simulink model "line_follower"  (R2020a)
settings: Solver=VariableStepAuto  StartTime=0.0  StopTime=70  RelTol=1e-3
InitFcn:
  | matlab_init
undefined symbols (not defined in the file or in its folder): A, A_double, A_s_double, A_s_single, A_single, Aaileron, Aelevator, Arudder, Athrust, B, B_double, B_s_double, B_s_single, B_single, Baileron, Belevator, Brudder, Bthrust, C, C_double, C_P, C_rollpitch, C_single, C_T, C_yaw, Caileron, Celevator, Crudder, Cthrust, D, D_double, D_single, Daileron, Delevator, DiscIntNeverNeededParam, Discrete, Drudder, Dthrust, g, I_flip, J, Jinv, K_a, K_e, K_r, K_t, L_double, L_single, measurement_noise, MotorMix, process_noise, Prop_H, q_single, r_single, tau2, Thrust_Sum, Time, trim_input, trim_state, Ts ... (+1)
libraries: simulink x5, ctrlSharedLib x5, vrlib x3, dspmtrx3 x1
(part 2 of 2)

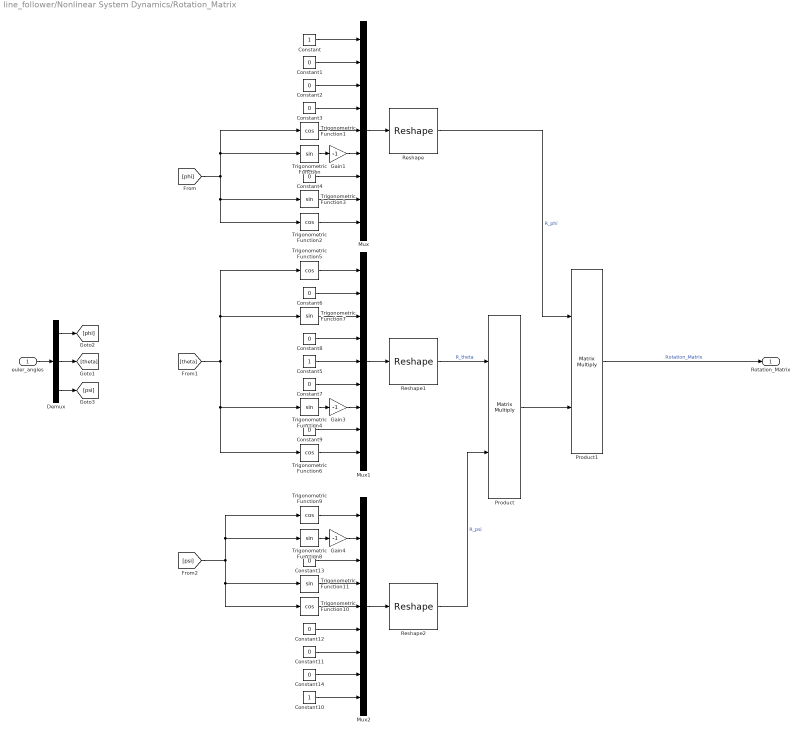
== system line_follower/Nonlinear System Dynamics/Rotation_Matrix ==
  "euler_angles " : Inport
  Constant : Constant
  Constant{1..4,6..9,11..14} (12 alike) : Constant  Value=0
  Constant10 : Constant
  Constant5 : Constant
  Demux : Demux  Outputs=3
  Gain1 : Gain  Gain=-1
  Gain3 : Gain  Gain=-1
  Gain4 : Gain  Gain=-1
  Mux : Mux  Inputs=9
  Mux1 : Mux  Inputs=9
  Mux2 : Mux  Inputs=9
  Product : Product  Multiplication=Matrix(*)
  Product1 : Product  Multiplication=Matrix(*)
  Reshape : Reshape  OutputDimensionality=Customize  OutputDimensions=[3,3]
  Reshape1 : Reshape  OutputDimensionality=Customize  OutputDimensions=[3,3]
  Reshape2 : Reshape  OutputDimensionality=Customize  OutputDimensions=[3,3]
  Trigonometric Function{,3..4,7..8,11} (6 alike) : Trigonometry
  Trigonometric Function{1..2,5..6,9..10} (6 alike) : Trigonometry  Operator=cos
  Rotation_Matrix : Outport
  wires:
  Constant9/1 -> Mux1/8
  Constant11/1 -> Mux2/7
  Trigonometric Function1/1 -> Mux/5
  Trigonometric Function3/1 -> Mux/8
  Constant5/1 -> Mux1/5
  Trigonometric Function7/1 -> Mux1/3
  Reshape/1 -> Product1/1  "R_phi"
  Mux1/1 -> Reshape1/1
  Trigonometric Function8/1 -> Gain4/1
  Constant7/1 -> Mux1/6
  Trigonometric Function2/1 -> Mux/9
  [phi] -> Trigonometric Function2/1, Trigonometric Function3/1, Trigonometric Function1/1, Trigonometric Function/1
  Trigonometric Function6/1 -> Mux1/9
  Constant12/1 -> Mux2/6
  Trigonometric Function4/1 -> Gain3/1
  [theta] -> Trigonometric Function7/1, Trigonometric Function5/1, Trigonometric Function4/1, Trigonometric Function6/1
  Reshape2/1 -> Product/2  "R_psi"
  Trigonometric Function/1 -> Gain1/1
  Product/1 -> Product1/2
  Trigonometric Function5/1 -> Mux1/1
  Trigonometric Function9/1 -> Mux2/1
  Mux/1 -> Reshape/1
  Constant/1 -> Mux/1
  Constant3/1 -> Mux/4
  Constant6/1 -> Mux1/2
  Mux2/1 -> Reshape2/1
  Constant2/1 -> Mux/3
  Constant1/1 -> Mux/2
  [psi] -> Trigonometric Function11/1, Trigonometric Function10/1, Trigonometric Function9/1, Trigonometric Function8/1
  Constant8/1 -> Mux1/4
  Constant4/1 -> Mux/7
  Constant13/1 -> Mux2/3
  Trigonometric Function11/1 -> Mux2/4
  Constant10/1 -> Mux2/9
  Reshape1/1 -> Product/1  "R_theta"
  Constant14/1 -> Mux2/8
  Trigonometric Function10/1 -> Mux2/5
  Product1/1 -> Rotation_Matrix/1  "Rotation_Matrix"
  Demux/3 -> [psi]
  Demux/2 -> [theta]
  "euler_angles "/1 -> Demux/1
  Demux/1 -> [phi]
  Gain3/1 -> Mux1/7
  Gain1/1 -> Mux/6
  Gain4/1 -> Mux2/2

== system line_follower/Toggle Controller/Hover ==
  Mux : Mux  Inputs=9
  p : Constant  Value=0
  phi : Constant  Value=0
  q : Constant  Value=0
  r : Constant  Value=0
  theta : Constant  Value=0
  u : Constant  Value=0
  v : Constant  Value=0
  w : Constant  Value=0
  z : Constant  Value=1.5
  Out1 : Outport
  wires:
  theta/1 -> Mux/8
  u/1 -> Mux/1
  p/1 -> Mux/5
  r/1 -> Mux/7
  z/1 -> Mux/4
  q/1 -> Mux/6
  phi/1 -> Mux/9
  w/1 -> Mux/3
  v/1 -> Mux/2
  Mux/1 -> Out1/1

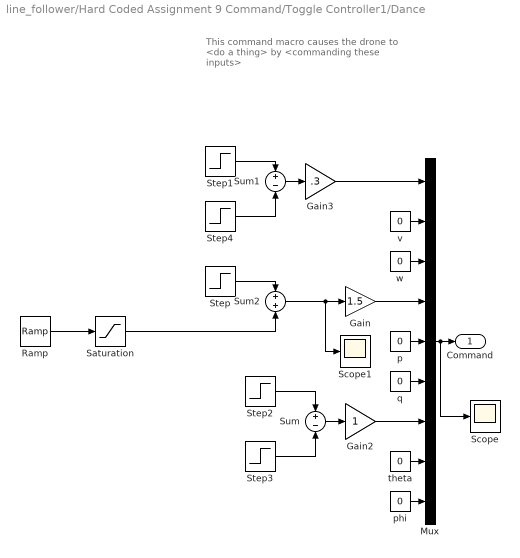
== system line_follower/Hard Coded Assignment 9 Command/Toggle Controller1/Dance ==
  note: This command macro causes the drone to <do a thing> by <commanding these inputs>
  Gain : Gain  Gain=1.5
  Gain2 : Gain
  Gain3 : Gain  Gain=.3
  Mux : Mux  Inputs=9
  Ramp : simulink/Sources/Ramp  slope=-.3  start=17  InitialOutput=0
  Saturation : Saturate  UpperLimit=1  LowerLimit=-1
  Scope : Scope
  Scope1 : Scope
  Step : Step  SampleTime=0
  Step1 : Step  Time=4  SampleTime=0
  Step2 : Step  Time=7  SampleTime=0
  Step3 : Step  Time=13.5  SampleTime=0
  Step4 : Step  Time=13.5  SampleTime=0
  Sum : Sum  Inputs=+-
  Sum1 : Sum  Inputs=+-
  Sum2 : Sum
  p : Constant  Value=0
  phi : Constant  Value=0
  q : Constant  Value=0
  theta : Constant  Value=0
  v : Constant  Value=0
  w : Constant  Value=0
  Command : Outport
  wires:
  Mux/1 -> Scope/1, Command/1
  theta/1 -> Mux/8
  p/1 -> Mux/5
  q/1 -> Mux/6
  v/1 -> Mux/2
  phi/1 -> Mux/9
  w/1 -> Mux/3
  Gain/1 -> Mux/4
  Step1/1 -> Sum1/1
  Step2/1 -> Sum/1
  Step3/1 -> Sum/2
  Sum/1 -> Gain2/1
  Gain2/1 -> Mux/7
  Sum1/1 -> Gain3/1
  Step4/1 -> Sum1/2
  Gain3/1 -> Mux/1
  Step/1 -> Sum2/1
  Sum2/1 -> Scope1/1, Gain/1
  Ramp/1 -> Saturation/1
  Saturation/1 -> Sum2/2

== system line_follower/Hard Coded Elevator Flip/Toggle Controller1/Hover ==
  Mux : Mux  Inputs=9
  p : Constant  Value=0
  phi : Constant  Value=0
  q : Constant  Value=0
  r : Constant  Value=0
  theta : Constant  Value=0
  u : Constant  Value=0
  v : Constant  Value=0
  w : Constant  Value=0
  z : Constant  Value=1.5
  Out1 : Outport
  wires:
  Mux/1 -> Out1/1
  v/1 -> Mux/2
  w/1 -> Mux/3
  phi/1 -> Mux/9
  q/1 -> Mux/6
  z/1 -> Mux/4
  r/1 -> Mux/7
  p/1 -> Mux/5
  u/1 -> Mux/1
  theta/1 -> Mux/8

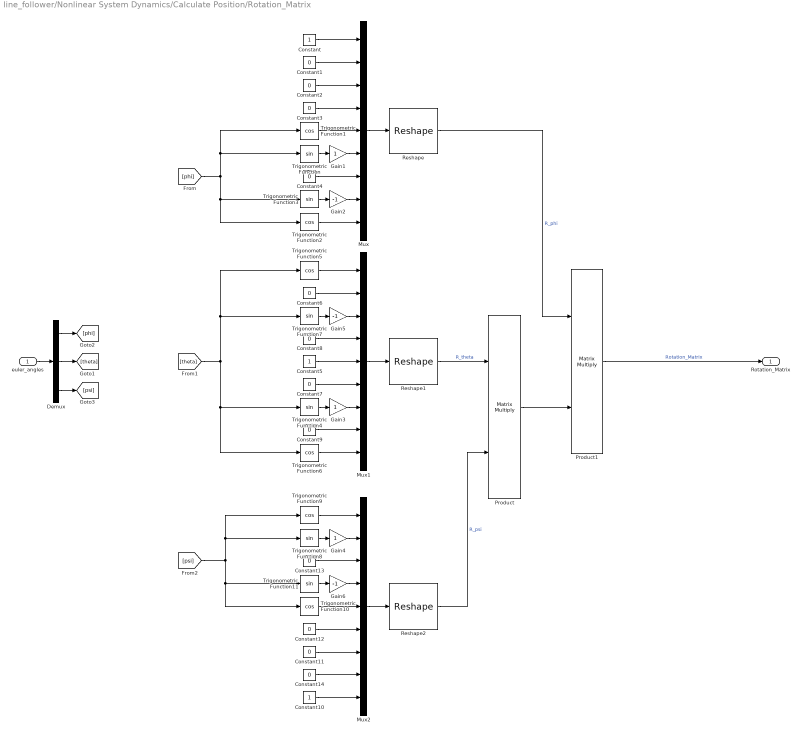
== system line_follower/Nonlinear System Dynamics/Calculate Position/Rotation_Matrix ==
  "euler_angles " : Inport
  Constant : Constant
  Constant{1..4,6..9,11..14} (12 alike) : Constant  Value=0
  Constant10 : Constant
  Constant5 : Constant
  Demux : Demux  Outputs=3
  Gain1 : Gain
  Gain2 : Gain  Gain=-1
  Gain3 : Gain
  Gain4 : Gain
  Gain5 : Gain  Gain=-1
  Gain6 : Gain  Gain=-1
  Mux : Mux  Inputs=9
  Mux1 : Mux  Inputs=9
  Mux2 : Mux  Inputs=9
  Product : Product  Multiplication=Matrix(*)
  Product1 : Product  Multiplication=Matrix(*)
  Reshape : Reshape  OutputDimensionality=Customize  OutputDimensions=[3,3]
  Reshape1 : Reshape  OutputDimensionality=Customize  OutputDimensions=[3,3]
  Reshape2 : Reshape  OutputDimensionality=Customize  OutputDimensions=[3,3]
  Trigonometric Function{,3..4,7..8,11} (6 alike) : Trigonometry
  Trigonometric Function{1..2,5..6,9..10} (6 alike) : Trigonometry  Operator=cos
  Rotation_Matrix : Outport
  wires:
  Constant9/1 -> Mux1/8
  Constant11/1 -> Mux2/7
  Trigonometric Function1/1 -> Mux/5
  Trigonometric Function3/1 -> Gain2/1
  Constant5/1 -> Mux1/5
  Trigonometric Function7/1 -> Gain5/1
  Reshape/1 -> Product1/1  "R_phi"
  Mux1/1 -> Reshape1/1
  Trigonometric Function8/1 -> Gain4/1
  Constant7/1 -> Mux1/6
  Trigonometric Function2/1 -> Mux/9
  [phi] -> Trigonometric Function2/1, Trigonometric Function3/1, Trigonometric Function1/1, Trigonometric Function/1
  Trigonometric Function6/1 -> Mux1/9
  Constant12/1 -> Mux2/6
  Trigonometric Function4/1 -> Gain3/1
  [theta] -> Trigonometric Function7/1, Trigonometric Function5/1, Trigonometric Function4/1, Trigonometric Function6/1
  Reshape2/1 -> Product/2  "R_psi"
  Trigonometric Function/1 -> Gain1/1
  Product/1 -> Product1/2
  Trigonometric Function5/1 -> Mux1/1
  Trigonometric Function9/1 -> Mux2/1
  Mux/1 -> Reshape/1
  Constant/1 -> Mux/1
  Constant3/1 -> Mux/4
  Constant6/1 -> Mux1/2
  Mux2/1 -> Reshape2/1
  Constant2/1 -> Mux/3
  Constant1/1 -> Mux/2
  [psi] -> Trigonometric Function11/1, Trigonometric Function10/1, Trigonometric Function9/1, Trigonometric Function8/1
  Constant8/1 -> Mux1/4
  Constant4/1 -> Mux/7
  Constant13/1 -> Mux2/3
  Trigonometric Function11/1 -> Gain6/1
  Constant10/1 -> Mux2/9
  Reshape1/1 -> Product/1  "R_theta"
  Constant14/1 -> Mux2/8
  Trigonometric Function10/1 -> Mux2/5
  Product1/1 -> Rotation_Matrix/1  "Rotation_Matrix"
  Demux/3 -> [psi]
  Demux/2 -> [theta]
  "euler_angles "/1 -> Demux/1
  Demux/1 -> [phi]
  Gain3/1 -> Mux1/7
  Gain1/1 -> Mux/6
  Gain4/1 -> Mux2/2
  Gain2/1 -> Mux/8
  Gain5/1 -> Mux1/3
  Gain6/1 -> Mux2/4

== system line_follower/Nonlinear System Dynamics/Calculate Velocity/Calculate_Thrust ==
  note: $F_{T} = \sum_{i=1}^4[0;0;C_{T}.*n.^2]$
  n : Inport
  Constant15 : Constant  Value=C_T(1)
  Constant16 : Constant  Value=2
  Gain4 : Gain  Gain=Thrust_Sum  Multiplication=Matrix(K*u)
      settings: AttributesFormatString=%<Gain>
  Gain5 : Gain  Gain=C_T(2)
  Power : Math  Operator=pow  SaturateOnIntegerOverflow=on
  Product2 : Product
  Sum1 : Sum  Inputs=++|
  F_T : Outport
  wires:
  Constant15/1 -> Sum1/1
  Gain4/1 -> F_T/1  "F_T"
  n/1 -> Power/1, Gain5/1
  Power/1 -> Product2/2  "props squared"
  Gain5/1 -> Sum1/2
  Sum1/1 -> Product2/1
  Product2/1 -> Gain4/1
  Constant16/1 -> Power/2

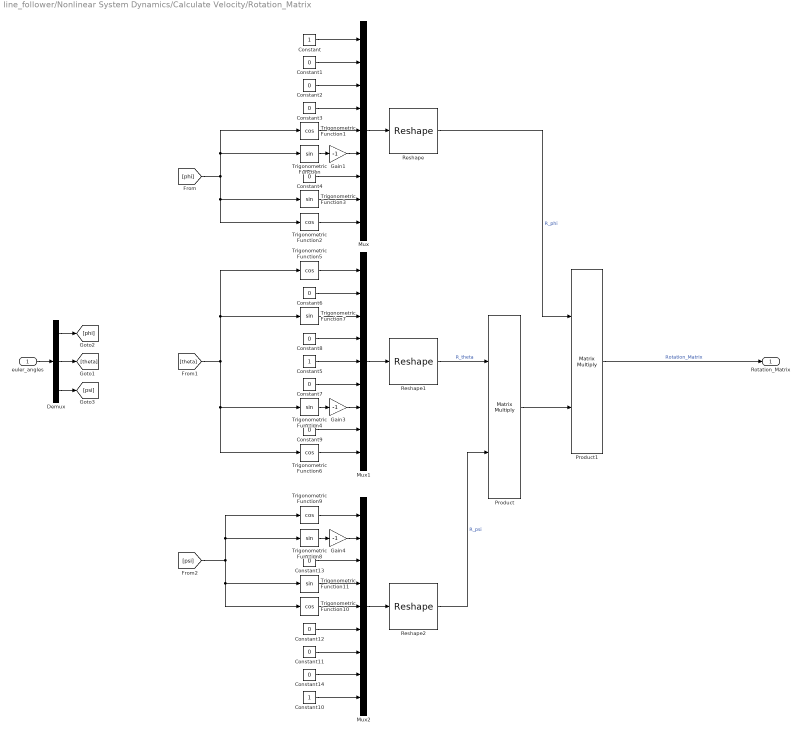
== system line_follower/Nonlinear System Dynamics/Calculate Velocity/Rotation_Matrix ==
  "euler_angles " : Inport
  Constant : Constant
  Constant{1..4,6..9,11..14} (12 alike) : Constant  Value=0
  Constant10 : Constant
  Constant5 : Constant
  Demux : Demux  Outputs=3
  Gain1 : Gain  Gain=-1
  Gain3 : Gain  Gain=-1
  Gain4 : Gain  Gain=-1
  Mux : Mux  Inputs=9
  Mux1 : Mux  Inputs=9
  Mux2 : Mux  Inputs=9
  Product : Product  Multiplication=Matrix(*)
  Product1 : Product  Multiplication=Matrix(*)
  Reshape : Reshape  OutputDimensionality=Customize  OutputDimensions=[3,3]
  Reshape1 : Reshape  OutputDimensionality=Customize  OutputDimensions=[3,3]
  Reshape2 : Reshape  OutputDimensionality=Customize  OutputDimensions=[3,3]
  Trigonometric Function{,3..4,7..8,11} (6 alike) : Trigonometry
  Trigonometric Function{1..2,5..6,9..10} (6 alike) : Trigonometry  Operator=cos
  Rotation_Matrix : Outport
  wires:
  Constant9/1 -> Mux1/8
  Constant11/1 -> Mux2/7
  Trigonometric Function1/1 -> Mux/5
  Trigonometric Function3/1 -> Mux/8
  Constant5/1 -> Mux1/5
  Trigonometric Function7/1 -> Mux1/3
  Reshape/1 -> Product1/1  "R_phi"
  Mux1/1 -> Reshape1/1
  Trigonometric Function8/1 -> Gain4/1
  Constant7/1 -> Mux1/6
  Trigonometric Function2/1 -> Mux/9
  [phi] -> Trigonometric Function2/1, Trigonometric Function3/1, Trigonometric Function1/1, Trigonometric Function/1
  Trigonometric Function6/1 -> Mux1/9
  Constant12/1 -> Mux2/6
  Trigonometric Function4/1 -> Gain3/1
  [theta] -> Trigonometric Function7/1, Trigonometric Function5/1, Trigonometric Function4/1, Trigonometric Function6/1
  Reshape2/1 -> Product/2  "R_psi"
  Trigonometric Function/1 -> Gain1/1
  Product/1 -> Product1/2
  Trigonometric Function5/1 -> Mux1/1
  Trigonometric Function9/1 -> Mux2/1
  Mux/1 -> Reshape/1
  Constant/1 -> Mux/1
  Constant3/1 -> Mux/4
  Constant6/1 -> Mux1/2
  Mux2/1 -> Reshape2/1
  Constant2/1 -> Mux/3
  Constant1/1 -> Mux/2
  [psi] -> Trigonometric Function11/1, Trigonometric Function10/1, Trigonometric Function9/1, Trigonometric Function8/1
  Constant8/1 -> Mux1/4
  Constant4/1 -> Mux/7
  Constant13/1 -> Mux2/3
  Trigonometric Function11/1 -> Mux2/4
  Constant10/1 -> Mux2/9
  Reshape1/1 -> Product/1  "R_theta"
  Constant14/1 -> Mux2/8
  Trigonometric Function10/1 -> Mux2/5
  Product1/1 -> Rotation_Matrix/1  "Rotation_Matrix"
  Demux/3 -> [psi]
  Demux/2 -> [theta]
  "euler_angles "/1 -> Demux/1
  Demux/1 -> [phi]
  Gain3/1 -> Mux1/7
  Gain1/1 -> Mux/6
  Gain4/1 -> Mux2/2

== matlab function line_follower/Control Design/Virtual Hough Transform Circle ==
  settings: updateMethod=DISCRETE  sampleTime=0.005
  data: y_cmd output; psi_cmd output; XY input
function [y_cmd, psi_cmd]= fcn(XY)

%% INIT X,Y to 0,2

x = XY(1);
y = XY(2);

path_rad = 2;

uav_rad = sqrt(x^2+y^2);
y_cmd = (uav_rad - path_rad);

path_angle = atan2(x,y);

if path_angle < -0.1
    path_angle = path_angle + 2*pi;
end

psi_cmd = (path_angle);

== matlab function line_follower/Drone Visualization ==
  data: T input
function drone_visualization(T)

%% /// IMPORTANT ///
%T is array that hold states
%ZED is pointing downwards
%MAKE A MATLAB FUNCTION BLOCK IN SIMULINK
%PASS IN THE NED STATES AND EULER ANGLES
%ADJUST THE STATES AS NECESSARY
%the drone is .18 meters by .18 meters

%the simulation will run MUCH slower while running the visualization
%you can comment out the function block to run the simulation quicker

%% constants
d = .18/2;
c1 = [d; d; 0]; %motor coordinates compared to center of drone
c2 = [d; -d; 0];
c3 = -c1;
c4 = -c2;

    %% adjust indices to get [X; Y; Z] and phi, theta, psi
    XYZ =  [T(1); ...
            T(2); ...
           -T(3)];
    phi =   T(7);
    theta = T(8);
    psi =   T(9);
    %%Defining rotation matrices
    Rx = [1 0 0; 0 cos(theta) sin(theta); 0 -sin(theta) cos(theta)];
    Ry = [cos(phi) 0 -sin(phi); 0 1 0; sin(phi) 0 cos(phi)];
    Rz = [cos(psi) sin(psi) 0; -sin(psi) cos(psi) 0; 0 0 1];
    b1 = Rz*Ry*Rx*c1;
    b2 = Rz*Ry*Rx*c2;
    b3 = Rz*Ry*Rx*c3;
    b4 = Rz*Ry*Rx*c4;
    m1 = XYZ + b1;
    m2 = XYZ + b2;
    m3 = XYZ + b3;
    m4 = XYZ + b4;
    P1 = [m1 m3];
    P2 = [m2 m4];
    P3 = [m1 m2];
    P4 = [m3 m4];

    %%displaying the drone
    plot3(P1(1,:),P1(2,:),P1(3,:),'k-', 'linewidth', 2);
    axis([-3 3 -3 3 -0 3]);
    xlabel('X Axis [Meters]')
    ylabel('Y Axis [Meters]')
    zlabel('Height [Meters]')
    hold on;
    grid on;
    plot3(P2(1,:),P2(2,:),P2(3,:),'k-', 'linewidth', 2);
    plot3(P3(1,:),P3(2,:),P3(3,:),'ob', 'linewidth', 1);
    plot3(P4(1,:),P4(2,:),P4(3,:),'ok', 'linewidth', 1);
    hold off
end

== matlab function line_follower/Control Design/Virtual Hough Transform Line ==
  settings: sampleTime=0.05
  data: y_cmd output; psi_cmd output; XY input
function [y_cmd, psi_cmd]= fcn(XY)

%% INIT X,Y to 0,2

x = XY(1);
y = XY(2);

a = 1;
b = 1;
c = -2;

% for line described by a*x+b*y+c=0
y_cmd = (a*x+b*y+c)/sqrt(a^2+b^2);

% path_rad = 2;
% 
% uav_rad = sqrt(x^2+y^2);
% y_cmd = (uav_rad - path_rad);

path_angle = atan2(a,b);

if path_angle < -0.1
    path_angle = path_angle + 2*pi;
end

psi_cmd = (path_angle);

== matlab function line_follower/Control Design/Virtual Hough Transform Angle ==
  settings: sampleTime=0.05
  data: y_cmd output; psi_cmd output; XY input
function [y_cmd, psi_cmd]= fcn(XY)

%% INIT X,Y to 0,2

x = XY(1);
y = XY(2);

a = 0;
b = 0;
c = 0;

if y > x
    a = 0;
    b = 1;
    c = -2;
else
    a = 1;
    b = 1/3;
    c = -2.66;
end

% for line described by a*x+b*y+c=0
y_cmd = (a*x+b*y+c)/sqrt(a^2+b^2);

% path_rad = 2;
% 
% uav_rad = sqrt(x^2+y^2);
% y_cmd = (uav_rad - path_rad);

path_angle = atan2(a,b);

if path_angle < -0.1
    path_angle = path_angle + 2*pi;
end

psi_cmd = (path_angle);

== matlab function line_follower/Control Design/Virtual Hough Transform All ==
  settings: sampleTime=0.05
  data: y_cmd output; psi_cmd output; XY input
function [y_cmd, psi_cmd]= fcn(XY)

%% INIT X,Y to -4,0

x = XY(1);
y = XY(2);

if x < -2
    a = -1;
    b = 1;
    c = -4;
    y_cmd = (a*x+b*y+c)/sqrt(a^2+b^2);
    path_angle = atan2(a,b);
elseif x < 2
    path_rad = sqrt(8);
    uav_rad = sqrt(x^2+y^2);
    y_cmd = (uav_rad - path_rad);
    path_angle = atan2(x,y);
else
    a = -1;
    b = 1;
    c = 0;
    y_cmd = (a*x+b*y+c)/sqrt(a^2+b^2);
    path_angle = atan2(a,b);
end


% if path_angle < -0.1
%     path_angle = path_angle + 2*pi;
% end

psi_cmd = (path_angle);
